simulink model "ESR_estimation"  (R2024b)
settings: Solver=ode3  StartTime=0.0  StopTime=1  FixedStep=4e-6  RelTol=1e-3
libraries: spsSeriesRLCBranchLib x10, spsCurrentMeasurementLib x4, spsIdealSwitchLib x4, spsVoltageMeasurementLib x3, spsGroundLib x2, spsLinearTransformerLib x2, spsDCVoltageSourceLib x1, spsDiodeLib x1, spsMeanLib x1, spsMosfetLib x1, dspstat3 x1, simulink x1
settings Model: Creator=Admin  LastModifiedBy=Admin

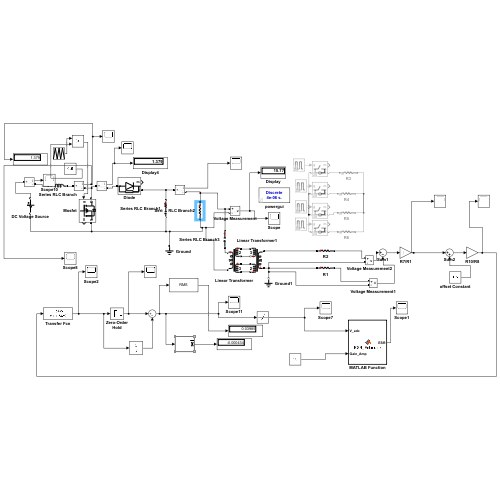
[thumbnail: Simulink's stored preview of the top-level diagram]
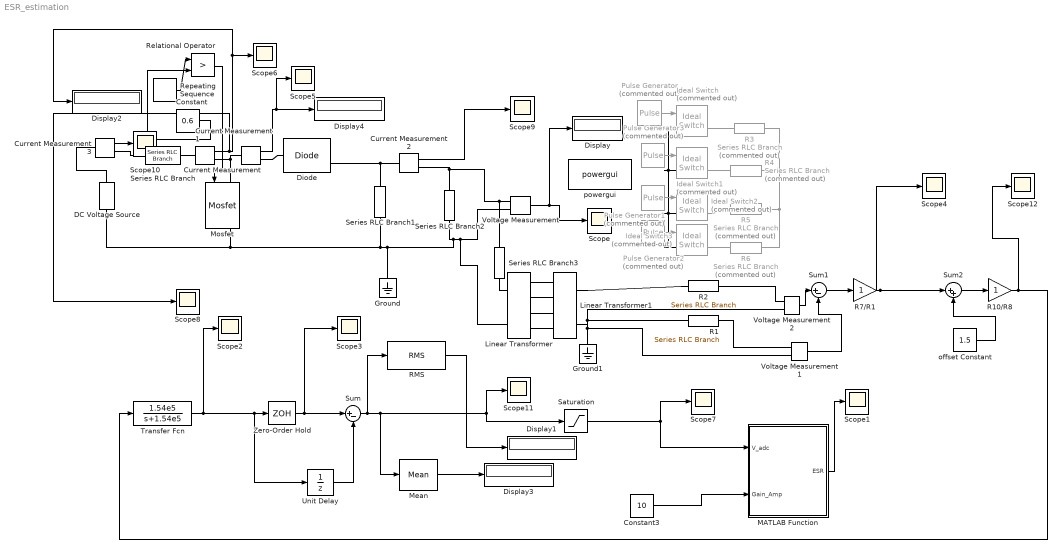
== system ESR_estimation ==
  Constant : Constant  Value=0.6
  Constant3 : Constant  Value=10
  Current Measurement{,1..3} (4 alike) : spsCurrentMeasurementLib/Current Measurement  PhasorSimulation=off  OutputType=Complex  PSBequivalent=0
  DC Voltage Source : spsDCVoltageSourceLib/DC Voltage Source  Amplitude=10  Measurements=None
  Diode : spsDiodeLib/Diode  Ron=0.001  Lon=0  Vf=0.8  IC=0  UseSnubber=0  Rs=500  Cs=250e-9  Measurements=on
  Display{,1..4} (5 alike) : Display
  Ground : spsGroundLib/Ground  LConnTagsString=a
  Ground1 : spsGroundLib/Ground  LConnTagsString=a
  Ideal Switch{,1..3} (4 alike) : spsIdealSwitchLib/Ideal Switch  Commented=on  Ron=0.001  Lon=0  IC=0  Rs=1e5  Cs=inf  Measurements=on
  Linear Transformer : spsLinearTransformerLib/Linear Transformer  UNITS=pu  NominalPower=[ 250e6 60 ]  winding1=[7.35e+05 0.002 0.08]  winding2=[3.15e+05 0.002 0.08]  ThreeWindings=on  winding3=[3.15e+05 0.002 0.08]  RmLm=[499.98 500]  Measurements=None  DataType=off
  Linear Transformer1 : spsLinearTransformerLib/Linear Transformer  UNITS=pu  NominalPower=[ 250e6 60 ]  winding1="[ 735e3  0.002  0.08 ]"  winding2="[ 315e3  0.002  0.08 ]"  ThreeWindings=on  winding3=[ 315e3 0.002 0.08 ]  RmLm=[ 500 500 ]  Measurements=None  DataType=off
  MATLAB Function : MATLAB Function  TreatAsAtomicUnit=on
  Mean : spsMeanLib/Mean  Freq=60  Vinit=0  Ts=0
  Mosfet : spsMosfetLib/Mosfet  Ron=0.1  Lon=0  Rd=0.01  Vfd=0  IC=0  Rs=1e5  Cs=1e-12  Measurements=on
  Pulse Generator : DiscretePulseGenerator  Commented=on  PulseType=Time based  Period=1/1000  PulseWidth=50
  Pulse Generator1 : DiscretePulseGenerator  Commented=on  PulseType=Time based  Period=1/10  PulseWidth=50  PhaseDelay=0.0005
  Pulse Generator2 : DiscretePulseGenerator  Commented=on  PulseType=Time based  Period=1/10  PulseWidth=50  PhaseDelay=0.00075
  Pulse Generator3 : DiscretePulseGenerator  Commented=on  PulseType=Time based  Period=1/1000  PulseWidth=50  PhaseDelay=0.0004
  R1 : spsSeriesRLCBranchLib/Series RLC Branch  LConnTagsString=__new0  RConnTagsString=__new0  BranchType=R  Resistance=500  Inductance=1e-3  SetiL0=off  InitialCurrent=0  Capacitance=1e-6  Setx0=off  InitialVoltage=0  Measurements=None
  R10/R8 : Gain
  R2 : spsSeriesRLCBranchLib/Series RLC Branch  LConnTagsString=__new0  RConnTagsString=__new0  BranchType=R  Resistance=5000  Inductance=1e-3  SetiL0=off  InitialCurrent=0  Capacitance=1e-6  Setx0=off  InitialVoltage=0  Measurements=None
  R3 : spsSeriesRLCBranchLib/Series RLC Branch  Commented=on  LConnTagsString=__new0  RConnTagsString=__new0  BranchType=R  Resistance=1000  Inductance=1e-3  SetiL0=off  InitialCurrent=0  Capacitance=1e-6  Setx0=off  InitialVoltage=0  Measurements=None
  R4 : spsSeriesRLCBranchLib/Series RLC Branch  Commented=on  LConnTagsString=__new0  RConnTagsString=__new0  BranchType=R  Resistance=2000  Inductance=1e-3  SetiL0=off  InitialCurrent=0  Capacitance=1e-6  Setx0=off  InitialVoltage=0  Measurements=None
  R5 : spsSeriesRLCBranchLib/Series RLC Branch  Commented=on  LConnTagsString=__new0  RConnTagsString=__new0  BranchType=R  Resistance=5000  Inductance=1e-3  SetiL0=off  InitialCurrent=0  Capacitance=1e-6  Setx0=off  InitialVoltage=0  Measurements=None
  R6 : spsSeriesRLCBranchLib/Series RLC Branch  Commented=on  LConnTagsString=__new0  RConnTagsString=__new0  BranchType=R  Resistance=10000  Inductance=1e-3  SetiL0=off  InitialCurrent=0  Capacitance=1e-6  Setx0=off  InitialVoltage=0  Measurements=None
  R7/R1 : Gain
  RMS : dspstat3/RMS  run=off  directionMode=Each column  dimension=1  InputProcessing=Columns as channels (frame based)  reset_popup=None
  Relational Operator : RelationalOperator  Operator=>  OutDataTypeStr=boolean  RndMeth=Simplest  InputSameDT=off
  Repeating Sequence : simulink/Sources/Repeating Sequence  rep_seq_t=[0 10e-6 20e-6]  rep_seq_y=[0 1 0]
  Saturation : Saturate  UpperLimit=5  LowerLimit=-5
  Scope{,1..12} (13 alike) : Scope
  Series RLC Branch : spsSeriesRLCBranchLib/Series RLC Branch  LConnTagsString=__new0  RConnTagsString=__new0  BranchType=L  Resistance=1  Inductance=220e-6  SetiL0=off  InitialCurrent=0  Capacitance=1e-6  Setx0=off  InitialVoltage=0  Measurements=None
  Series RLC Branch1 : spsSeriesRLCBranchLib/Series RLC Branch  LConnTagsString=__new0  RConnTagsString=__new0  BranchType=RC  Resistance=0.1  Inductance=1e-3  SetiL0=off  InitialCurrent=0  Capacitance=100e-6  Setx0=off  InitialVoltage=0  Measurements=None
  Series RLC Branch2 : spsSeriesRLCBranchLib/Series RLC Branch  LConnTagsString=__new0  RConnTagsString=__new0  BranchType=R  Resistance=20  Inductance=1e-3  SetiL0=off  InitialCurrent=0  Capacitance=1e-6  Setx0=off  InitialVoltage=0  Measurements=None
  Series RLC Branch3 : spsSeriesRLCBranchLib/Series RLC Branch  LConnTagsString=__new0  RConnTagsString=__new0  BranchType=C  Resistance=1  Inductance=1e-3  SetiL0=off  InitialCurrent=0  Capacitance=10e-6  Setx0=off  InitialVoltage=0  Measurements=None
  Sum : Sum  Inputs=|+-
  Sum1 : Sum  Inputs=|+-
  Sum2 : Sum  Inputs=|++
  Transfer Fcn : TransferFcn  Numerator=[1.54e5]  Denominator=[1 1.54e5]
  Unit Delay : UnitDelay  SampleTime=4e-6  HasFrameUpgradeWarning=on
  Voltage Measurement : spsVoltageMeasurementLib/Voltage Measurement  PhasorSimulation=off  OutputType=Complex  PSBequivalent=0
  Voltage Measurement1 : spsVoltageMeasurementLib/Voltage Measurement  PhasorSimulation=off  OutputType=Complex  PSBequivalent=0
  Voltage Measurement2 : spsVoltageMeasurementLib/Voltage Measurement  PhasorSimulation=off  OutputType=Complex  PSBequivalent=0
  Zero-Order Hold : ZeroOrderHold  SampleTime=4e-6
  offset Constant : Constant  Value=1.5
  powergui : sps_lib/powergui  Priority=1  SimulationMode=Discrete  SampleTime=4e-6  frequency=60  Iterations=50  frequencyindice=0  Pbase=100e6  ErrMax=1e-4  UnitsV=kV  UnitsW=MW  buscounter=0  FunctionMessages=off  echomessages=off  EnableUseOfTLC=off  CurrentSourceSwitches=off  DisableSnubberDevices=off  DisableRonSwitches=off  DisableVfSwitches=off  DisplayEquations=off  AutomaticDiscreteSolvers=off  SolverType=Tustin/Backward Euler (TBE)  Interpol=off  ExternalGateDelay=off  methode=off  Ts=100  x0status=blocks  SPID=on  SwTol=0  HookPort=off  NonlinearTolerance=1e-4  nMaxIteration=100  ContinueOnMaxIteration=off  RestoreLinks=warning  ResistiveCurrentMeasurement=off  Frange=[0:2:500]  Ylog=off  Xlog=on  ShowGrid=off  save=off  variable=ZData  structure=0  ZoomFFT=off  StartTime=0.0  cycles=1  DisplayStyle=1  fundamental=60  FreqAxis=off  MaxFrequency=1000  frequencyindicesteady=1  RmsSteady=1  display=off
  wires:
  Voltage Measurement/1 -> Scope/1, Display/1
  R7/R1/1 -> Sum2/1, Scope4/1
  Sum2/1 -> R10/R8/1
  MATLAB Function/1(ESR) -> Scope1/1
  offset Constant/1 -> Sum2/2
  Transfer Fcn/1 -> Unit Delay/1, Zero-Order Hold/1, Scope2/1
  Pulse Generator/1 -> Ideal Switch/1
  Pulse Generator2/1 -> Ideal Switch3/1
  Pulse Generator1/1 -> Ideal Switch2/1
  Pulse Generator3/1 -> Ideal Switch1/1
  Current Measurement/1 -> Scope5/1, Display4/1
  Current Measurement1/1 -> Scope8/1, Display2/1, Scope6/1
  Relational Operator/1 -> Mosfet/1
  Repeating Sequence/1 -> Relational Operator/1
  Constant/1 -> Relational Operator/2
  Current Measurement2/1 -> Scope9/1
  Current Measurement3/1 -> Scope10/1
  Zero-Order Hold/1 -> Scope3/1, Sum/1
  Sum/1 -> RMS/1, Mean/1, Saturation/1, Scope11/1
  Voltage Measurement1/1 -> Sum1/2
  Voltage Measurement2/1 -> Sum1/1
  Unit Delay/1 -> Sum/2
  Sum1/1 -> R7/R1/1
  R10/R8/1 -> Transfer Fcn/1, Scope12/1
  Constant3/1 -> MATLAB Function/2(Gain_Amp)
  Saturation/1 -> Scope7/1, MATLAB Function/1(V_adc)
  RMS/1 -> Display1/1
  Mean/1 -> Display3/1
  connections:
  Current Measurement/LConn1 -- Current Measurement1/RConn1 -- Mosfet/LConn1
  Ground/LConn1 -- Linear Transformer/LConn2 -- Voltage Measurement/LConn2 -- Series RLC Branch2/RConn1 -- Series RLC Branch1/RConn1 -- DC Voltage Source/LConn1 -- Mosfet/RConn1
  Series RLC Branch3/LConn1 -- Series RLC Branch2/LConn1 -- Current Measurement2/RConn1 -- Voltage Measurement/LConn1
  Linear Transformer/RConn1 -- Linear Transformer1/RConn4
  Linear Transformer/RConn2 -- Linear Transformer1/RConn3
  Linear Transformer/RConn3 -- Linear Transformer1/RConn2
  Linear Transformer/RConn4 -- Linear Transformer1/RConn1
  Series RLC Branch3/RConn1 -- Linear Transformer/LConn1
  Ground1/LConn1 -- R1/LConn1 -- Voltage Measurement2/LConn2 -- Linear Transformer1/LConn1 -- Voltage Measurement1/LConn2
  Ideal Switch3/LConn1 -- Ideal Switch2/LConn1 -- Ideal Switch1/LConn1 -- Ideal Switch/LConn1
  Ideal Switch/RConn1 -- R3/LConn1
  Ideal Switch1/RConn1 -- R4/LConn1
  R5/LConn1 -- Ideal Switch2/RConn1
  R6/LConn1 -- Ideal Switch3/RConn1
  Current Measurement/RConn1 -- Diode/LConn1
  Current Measurement1/LConn1 -- Series RLC Branch/RConn1
  Diode/RConn1 -- Current Measurement2/LConn1 -- Series RLC Branch1/LConn1
  DC Voltage Source/RConn1 -- Current Measurement3/LConn1
  Series RLC Branch/LConn1 -- Current Measurement3/RConn1
  R3/RConn1 -- R4/RConn1 -- R6/RConn1 -- R5/RConn1
  R1/RConn1 -- Voltage Measurement1/LConn1
  Linear Transformer1/LConn2 -- R2/LConn1
  R2/RConn1 -- Voltage Measurement2/LConn1

== matlab function ESR_estimation/MATLAB Function ==
  data: V_adc input; ESR output; Gain_Amp input
function ESR = ESR_Estimator(V_adc, Gain_Amp)

persistent ESR_filt

if isempty(ESR_filt)
    ESR_filt = 0;
end

I_CAP_STEP = 0.3;

K = 10;

ESR_inst = (K * abs(V_adc)) / (Gain_Amp * I_CAP_STEP);

alpha = 0.05;
ESR_filt = alpha * ESR_inst + (1 - alpha) * ESR_filt;

ESR = ESR_filt;

end
